simulink model "nomotofirstorder"  (R2017b)
settings: Solver=VariableStepAuto  StartTime=0.0  StopTime=tstop  RelTol=1e-3
values from neighbouring files (symbols this model uses):
  amp = -0.3    [run18.m]
  omega_d = 0.008    [run18.m]
  tsamp = 10    [run18.m]    (also in run18_plot.m)
  x = lsqcurvefit(F,x0, tdata, rdata)    [run_task_1_2.m]
settings Model: Creator=henningward  LastModifiedBy=henningward
settings CodeAppCC: StateflowObjectComments=on

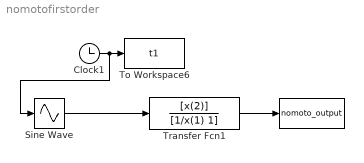
== system nomotofirstorder ==
  " " : ToWorkspace  VariableName=nomoto_output  SampleTime=-1
  Clock1 : Clock
  Sine Wave : Sin  TimeSource=Use external signal  Amplitude=amp  Frequency=omega_d  SampleTime=0
  To Workspace6 : ToWorkspace  VariableName=t1  SampleTime=tsamp
  Transfer Fcn1 : TransferFcn  Numerator=[x(2)]  Denominator=[1/x(1) 1]
  wires:
  Transfer Fcn1/1 -> " "/1
  Clock1/1 -> Sine Wave/1, To Workspace6/1
  Sine Wave/1 -> Transfer Fcn1/1
